simulink model "Model_Comparison"  (R2021a)
settings: Solver=VariableStepAuto  StartTime=0.0  StopTime=3600  RelTol=1e-3
undefined symbols (not defined in the file): A_cell, C1_LUT, Capacity_LUT, Cp_cell, H_cell, M_cell, OCV_LUT, R0_LUT, R1_LUT, SOC_LUT, T_amb, Temperature_LUT
libraries: simulink x1
settings Model: Creator=gopin  LastModifiedBy=gopin

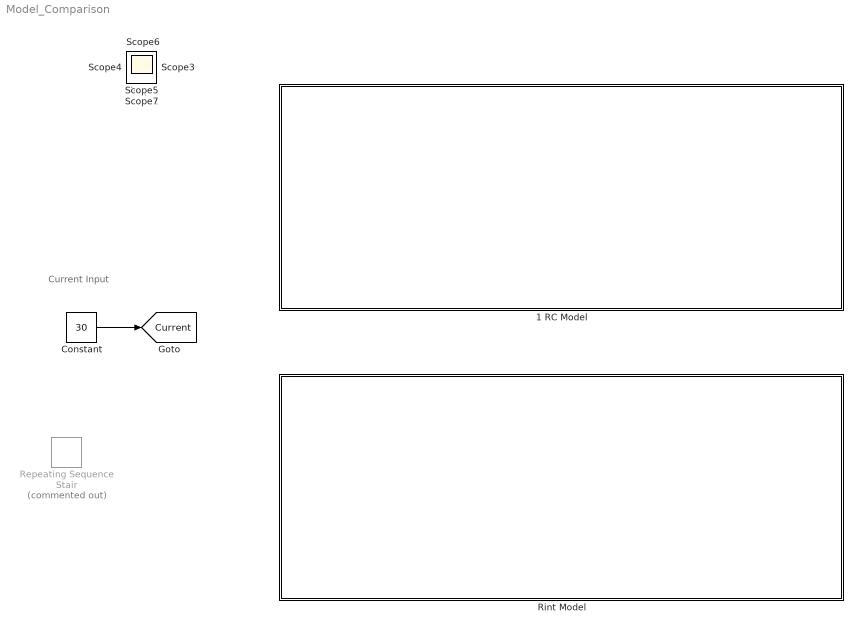
== system Model_Comparison ==
  note: Current Input
  1 RC Model : Subsystem
  Constant : Constant  Value=30
  Repeating Sequence Stair : simulink/Sources/Repeating Sequence Stair  Commented=on  OutValues=[0 0 0 5 9 15 18 18 18 11 8 3 1]  tsamp=-1  OutMin=[]  OutMax=[]  OutDataTypeStr=double  OutputDataTypeScalingMode=double  OutDataType=fixdt(0,8)  ConRadixGroup=Best Precision: Vector-wise  OutScaling=2^-12
  Rint Model : Subsystem
  Scope{,1..7} (8 alike) : Scope
  tag scope: Current=global
  wires:
  Constant/1 -> [Current]

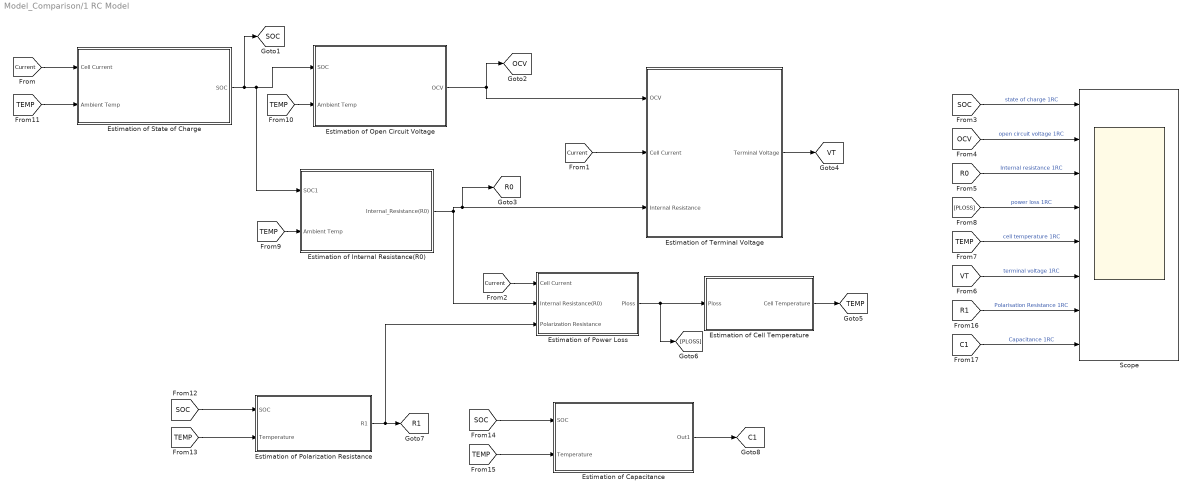
== system Model_Comparison/1 RC Model ==
  Estimation of Capacitance : Subsystem
  Estimation of Cell Temperature : Subsystem
  Estimation of Internal Resistance(R0) : Subsystem
  Estimation of Open Circuit Voltage : Subsystem
  Estimation of Polarization Resistance : Subsystem
  Estimation of Power Loss : Subsystem
  "Estimation of State of Charge " : Subsystem
  Estimation of Terminal Voltage : Subsystem
  Scope : Scope  NumInputPorts=8
  tag scope: C1=global, OCV=global, R0=global, R1=global, SOC=global, TEMP=global, VT=global
  wires:
  Estimation of Terminal Voltage/1(Terminal Voltage) -> [VT]
  [SOC] -> Estimation of Polarization Resistance/1(SOC)
  Estimation of Capacitance/1(Out1) -> [C1]
  [PLOSS] -> Scope/4  "power loss 1RC"
  Estimation of Power Loss/1(Ploss) -> [PLOSS], Estimation of Cell Temperature/1(Ploss)
  [SOC] -> Estimation of Capacitance/1(SOC)
  Estimation of Internal Resistance(R0)/1(Internal_Resistance(R0)) -> [R0], Estimation of Terminal Voltage/3(Internal Resistance), Estimation of Power Loss/2(Internal Resistance(R0))
  [OCV] -> Scope/2  "open circuit voltage 1RC"
  [VT] -> Scope/6  "terminal voltage 1RC"
  [SOC] -> Scope/1  "state of charge 1RC"
  [TEMP] -> Scope/5  "cell temperature 1RC"
  [TEMP] -> Estimation of Capacitance/2(Temperature)
  Estimation of Polarization Resistance/1(R1) -> Estimation of Power Loss/3(Polarization Resistance), [R1]
  [TEMP] -> Estimation of Polarization Resistance/2(Temperature)
  [Current] -> Estimation of Terminal Voltage/2(Cell Current)
  "Estimation of State of Charge "/1(SOC) -> [SOC], Estimation of Internal Resistance(R0)/1(SOC1), Estimation of Open Circuit Voltage/1(SOC)
  Estimation of Open Circuit Voltage/1(OCV) -> Estimation of Terminal Voltage/1(OCV), [OCV]
  [Current] -> Estimation of Power Loss/1(Cell Current)
  [R0] -> Scope/3  "Internal resistance 1RC"
  [TEMP] -> Estimation of Open Circuit Voltage/2(Ambient Temp)
  [Current] -> "Estimation of State of Charge "/1(Cell Current)
  [TEMP] -> Estimation of Internal Resistance(R0)/2(Ambient Temp)
  [TEMP] -> "Estimation of State of Charge "/2(Ambient Temp)
  Estimation of Cell Temperature/1(Cell Temperature) -> [TEMP]
  [R1] -> Scope/7  "Polarisation Resistance 1RC"
  [C1] -> Scope/8  "Capacitance 1RC"

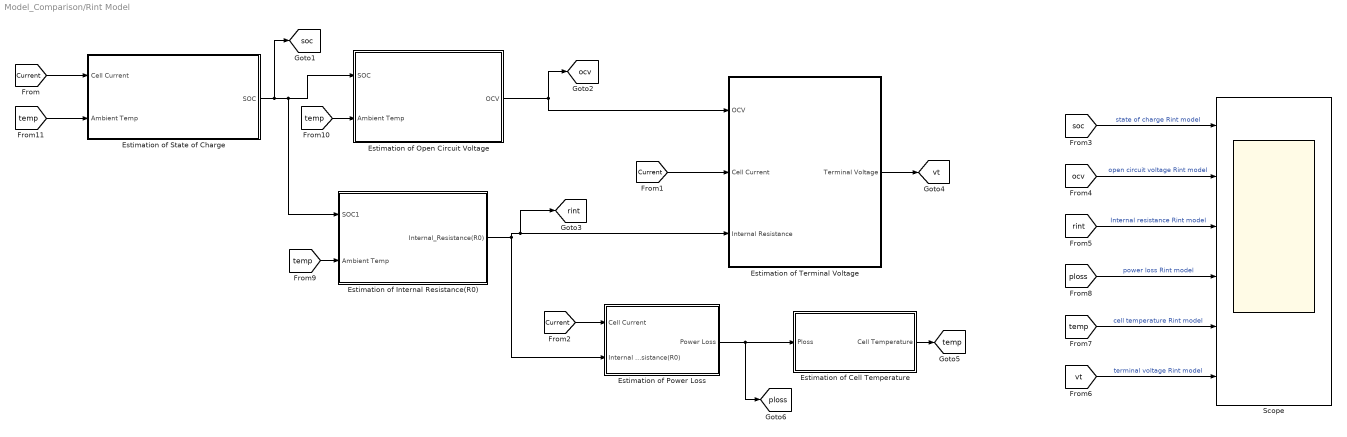
== system Model_Comparison/Rint Model ==
  Estimation of Cell Temperature : Subsystem
  Estimation of Internal Resistance(R0) : Subsystem
  Estimation of Open Circuit Voltage : Subsystem
  Estimation of Power Loss : Subsystem
  "Estimation of State of Charge " : Subsystem
  Estimation of Terminal Voltage : Subsystem
  Scope : Scope  NumInputPorts=6
  tag scope: ocv=global, ploss=global, rint=global, soc=global, temp=global, vt=global
  wires:
  [temp] -> "Estimation of State of Charge "/2(Ambient Temp)
  "Estimation of State of Charge "/1(SOC) -> [soc], Estimation of Internal Resistance(R0)/1(SOC1), Estimation of Open Circuit Voltage/1(SOC)
  [temp] -> Estimation of Internal Resistance(R0)/2(Ambient Temp)
  Estimation of Power Loss/1(Power Loss) -> [ploss], Estimation of Cell Temperature/1(Ploss)
  [Current] -> Estimation of Power Loss/1(Cell Current)
  [rint] -> Scope/3  "Internal resistance Rint model"
  [ocv] -> Scope/2  "open circuit voltage Rint model"
  [temp] -> Scope/5  "cell temperature Rint model"
  [ploss] -> Scope/4  "power loss Rint model"
  Estimation of Cell Temperature/1(Cell Temperature) -> [temp]
  [Current] -> "Estimation of State of Charge "/1(Cell Current)
  Estimation of Internal Resistance(R0)/1(Internal_Resistance(R0)) -> [rint], Estimation of Terminal Voltage/3(Internal Resistance), Estimation of Power Loss/2(Internal Resistance(R0))
  [Current] -> Estimation of Terminal Voltage/2(Cell Current)
  Estimation of Open Circuit Voltage/1(OCV) -> Estimation of Terminal Voltage/1(OCV), [ocv]
  Estimation of Terminal Voltage/1(Terminal Voltage) -> [vt]
  [vt] -> Scope/6  "terminal voltage Rint model"
  [temp] -> Estimation of Open Circuit Voltage/2(Ambient Temp)
  [soc] -> Scope/1  "state of charge Rint model"

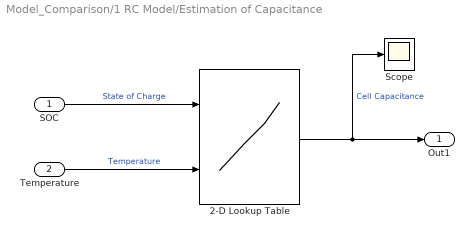
== system Model_Comparison/1 RC Model/Estimation of Capacitance ==
  SOC : Inport
  Temperature : Inport  Port=2
  2-D Lookup Table : Lookup_n-D  BreakpointsForDimension1=SOC_LUT  BreakpointsForDimension2=Temperature_LUT  Table=C1_LUT  InternalRulePriority=Speed  RndMeth=Simplest  InputSameDT=on
      settings: InputPortMap=u0,u1
  Scope : Scope
  Out1 : Outport
  wires:
  SOC/1 -> 2-D Lookup Table/1  "State of Charge"
  Temperature/1 -> 2-D Lookup Table/2  "Temperature"
  2-D Lookup Table/1 -> Scope/1, Out1/1  "Cell Capacitance"

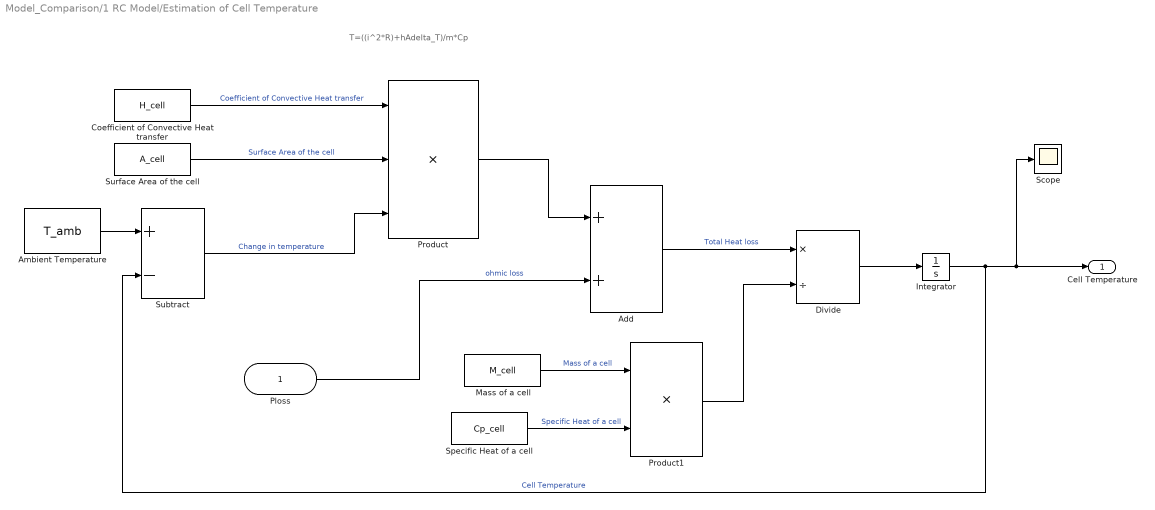
== system Model_Comparison/1 RC Model/Estimation of Cell Temperature ==
  note: T=((i^2*R)+hAdelta_T)/m*Cp
  Ploss : Inport
  Add : Sum
  Ambient Temperature : Constant  Value=T_amb
  Coefficient of Convective Heat transfer : Constant  Value=H_cell
  Divide : Product  Inputs=*/
  Integrator : Integrator  InitialCondition=T_amb  UpperSaturationLimit=353.15  LowerSaturationLimit=T_amb
  Mass of a cell : Constant  Value=M_cell
  Product : Product  Inputs=3
  Product1 : Product
  Scope : Scope
  Specific Heat of a cell : Constant  Value=Cp_cell
  Subtract : Sum  Inputs=+-
  Surface Area of the cell : Constant  Value=A_cell
  Cell Temperature : Outport
  wires:
  Ambient Temperature/1 -> Subtract/1
  Coefficient of Convective Heat transfer/1 -> Product/1  "Coefficient of Convective Heat transfer"
  Surface Area of the cell/1 -> Product/2  "Surface Area of the cell"
  Subtract/1 -> Product/3  "Change in temperature"
  Product/1 -> Add/1
  Ploss/1 -> Add/2  "ohmic loss"
  Add/1 -> Divide/1  "Total Heat loss"
  Product1/1 -> Divide/2
  Mass of a cell/1 -> Product1/1  "Mass of a cell"
  Specific Heat of a cell/1 -> Product1/2  "Specific Heat of a cell"
  Divide/1 -> Integrator/1
  Integrator/1 -> Subtract/2, Scope/1, Cell Temperature/1  "Cell Temperature"

== system Model_Comparison/1 RC Model/Estimation of Internal Resistance(R0) ==
  SOC1 : Inport
  Ambient Temp : Inport  Port=2
  2-D Lookup Table1 : Lookup_n-D  BreakpointsForDimension1=SOC_LUT  BreakpointsForDimension2=Temperature_LUT  Table=R0_LUT  InternalRulePriority=Speed  RndMeth=Simplest  InputSameDT=on
      settings: InputPortMap=u0,u1
  Scope : Scope
  Internal_Resistance(R0) : Outport
  wires:
  SOC1/1 -> 2-D Lookup Table1/1  "state of charge"
  2-D Lookup Table1/1 -> Scope/1, Internal_Resistance(R0)/1  "Internal Resistance"
  Ambient Temp/1 -> 2-D Lookup Table1/2  "Ambient Temperature"

== system Model_Comparison/1 RC Model/Estimation of Open Circuit Voltage ==
  SOC : Inport
  Ambient Temp : Inport  Port=2
  2-D Lookup Table : Lookup_n-D  BreakpointsForDimension1=SOC_LUT  BreakpointsForDimension2=Temperature_LUT  Table=OCV_LUT  InternalRulePriority=Speed  RndMeth=Simplest  InputSameDT=on
      settings: InputPortMap=u0,u1
  Scope : Scope
  OCV : Outport
  wires:
  SOC/1 -> 2-D Lookup Table/1  "state of charge"
  2-D Lookup Table/1 -> Scope/1, OCV/1  "open circuit voltage"
  Ambient Temp/1 -> 2-D Lookup Table/2  "Ambient Temperature"

== system Model_Comparison/1 RC Model/Estimation of Polarization Resistance ==
  SOC : Inport
  Temperature : Inport  Port=2
  2-D Lookup Table : Lookup_n-D  BreakpointsForDimension1=SOC_LUT  BreakpointsForDimension2=Temperature_LUT  Table=R1_LUT  InternalRulePriority=Speed  RndMeth=Simplest  InputSameDT=on
      settings: InputPortMap=u0,u1
  Scope : Scope
  R1 : Outport
  wires:
  SOC/1 -> 2-D Lookup Table/1  "State of Charge"
  Temperature/1 -> 2-D Lookup Table/2  "Temperature"
  2-D Lookup Table/1 -> Scope/1, R1/1  "Polarization Resistance"

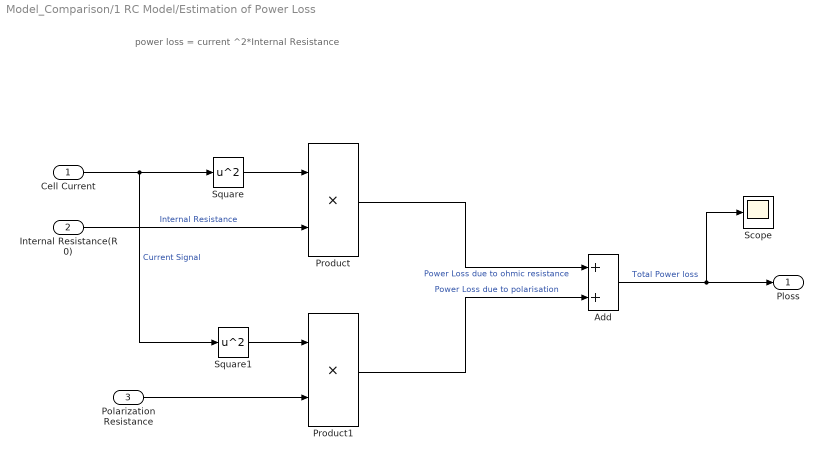
== system Model_Comparison/1 RC Model/Estimation of Power Loss ==
  note: power loss = current ^2*Internal Resistance
  Cell Current : Inport
  Internal Resistance(R0) : Inport  Port=2
  Polarization Resistance : Inport  Port=3
  Add : Sum
  Product : Product
  Product1 : Product
  Scope : Scope
  Square : Math  Operator=square  SaturateOnIntegerOverflow=on
  Square1 : Math  Operator=square  SaturateOnIntegerOverflow=on
  Ploss : Outport
  wires:
  Cell Current/1 -> Square1/1, Square/1  "Current Signal"
  Square/1 -> Product/1
  Product/1 -> Add/1  "Power Loss due to ohmic resistance"
  Internal Resistance(R0)/1 -> Product/2  "Internal Resistance"
  Square1/1 -> Product1/1
  Polarization Resistance/1 -> Product1/2
  Product1/1 -> Add/2  "Power Loss due to polarisation"
  Add/1 -> Scope/1, Ploss/1  "Total Power loss"

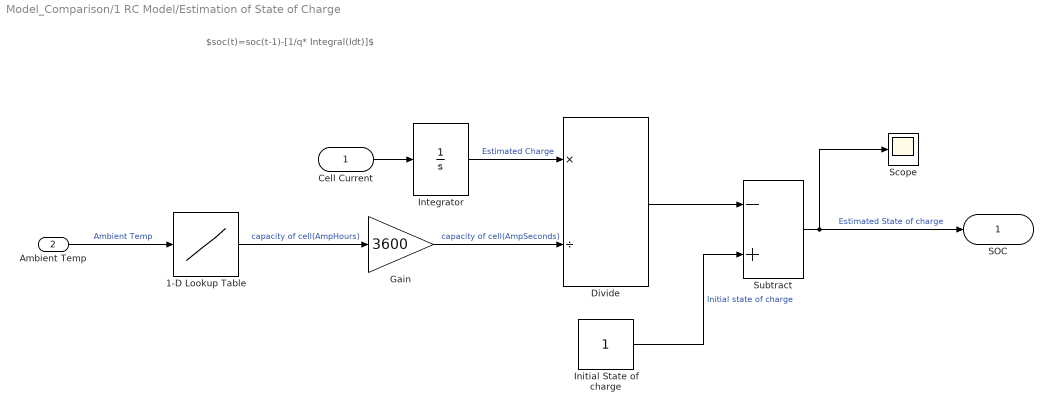
== system Model_Comparison/1 RC Model/Estimation of State of Charge  ==
  note: $soc(t)=soc(t-1)-[1/q* Integral(Idt)]$
  Cell Current : Inport
  Ambient Temp : Inport  Port=2
  1-D Lookup Table : Lookup_n-D  NumberOfTableDimensions=1  BreakpointsForDimension1=Temperature_LUT  Table=Capacity_LUT  InternalRulePriority=Speed  RndMeth=Simplest  InputSameDT=on
  Divide : Product  Inputs=*/
  Gain : Gain  Gain=3600
  Initial State of charge : Constant
  Integrator : Integrator
  Scope : Scope
  Subtract : Sum  Inputs=-+
  SOC : Outport
  wires:
  Initial State of charge/1 -> Subtract/2  "Initial state of charge"
  Subtract/1 -> Scope/1, SOC/1  "Estimated State of charge"
  Integrator/1 -> Divide/1  "Estimated Charge"
  Divide/1 -> Subtract/1
  Cell Current/1 -> Integrator/1
  1-D Lookup Table/1 -> Gain/1  "capacity of cell(AmpHours)"
  Gain/1 -> Divide/2  "capacity of cell(AmpSeconds)"
  Ambient Temp/1 -> 1-D Lookup Table/1  "Ambient Temp"

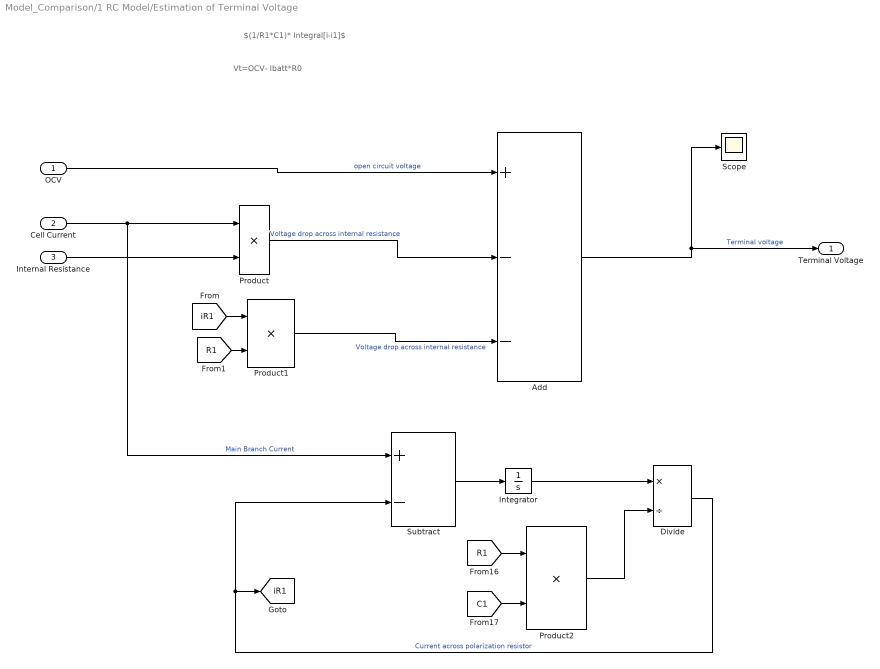
== system Model_Comparison/1 RC Model/Estimation of Terminal Voltage ==
  note: Vt=OCV- Ibatt*R0
  note: $(1/R1*C1)* Integral[i-i1]$
  OCV : Inport
  Cell Current : Inport  Port=2
  Internal Resistance : Inport  Port=3
  Add : Sum  Inputs=+--
  Divide : Product  Inputs=*/
  Integrator : Integrator
  Product : Product
  Product1 : Product
  Product2 : Product
  Scope : Scope
  Subtract : Sum  Inputs=+-
  Terminal Voltage : Outport
  tag scope: iR1=global
  wires:
  Add/1 -> Scope/1, Terminal Voltage/1  "Terminal voltage"
  OCV/1 -> Add/1  "open circuit voltage"
  Product/1 -> Add/2  "Voltage drop across internal resistance"
  Cell Current/1 -> Subtract/1, Product/1  "Main Branch Current"
  Internal Resistance/1 -> Product/2
  Product1/1 -> Add/3  "Voltage drop across internal resistance"
  Divide/1 -> [iR1], Subtract/2  "Current across polarization resistor"
  Subtract/1 -> Integrator/1
  Integrator/1 -> Divide/1
  Product2/1 -> Divide/2
  [R1] -> Product2/1
  [C1] -> Product2/2
  [iR1] -> Product1/1
  [R1] -> Product1/2

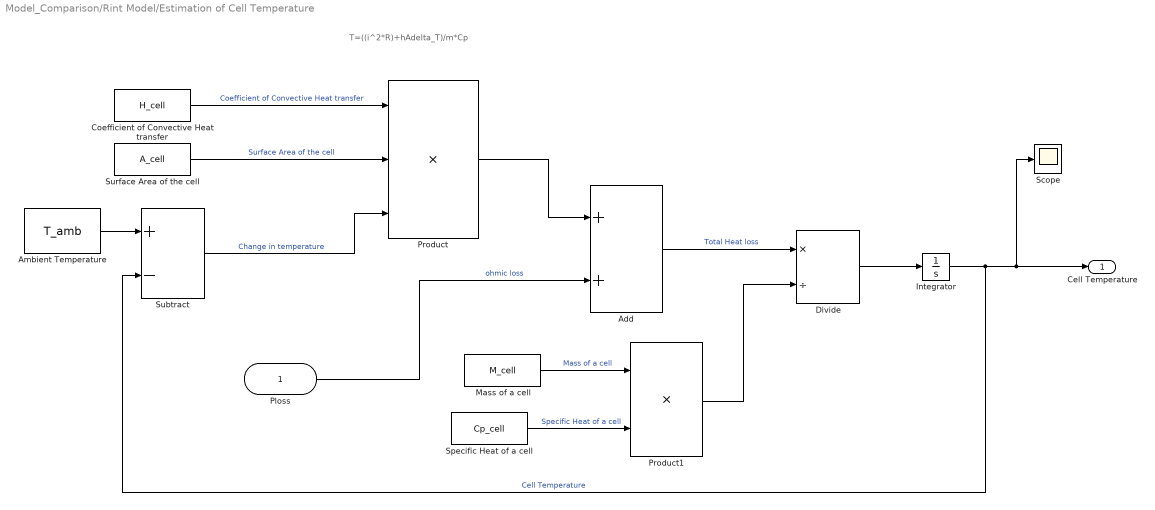
== system Model_Comparison/Rint Model/Estimation of Cell Temperature ==
  note: T=((i^2*R)+hAdelta_T)/m*Cp
  Ploss : Inport
  Add : Sum
  Ambient Temperature : Constant  Value=T_amb
  Coefficient of Convective Heat transfer : Constant  Value=H_cell
  Divide : Product  Inputs=*/
  Integrator : Integrator  InitialCondition=T_amb  UpperSaturationLimit=353.15  LowerSaturationLimit=T_amb
  Mass of a cell : Constant  Value=M_cell
  Product : Product  Inputs=3
  Product1 : Product
  Scope : Scope
  Specific Heat of a cell : Constant  Value=Cp_cell
  Subtract : Sum  Inputs=+-
  Surface Area of the cell : Constant  Value=A_cell
  Cell Temperature : Outport
  wires:
  Ambient Temperature/1 -> Subtract/1
  Coefficient of Convective Heat transfer/1 -> Product/1  "Coefficient of Convective Heat transfer"
  Surface Area of the cell/1 -> Product/2  "Surface Area of the cell"
  Subtract/1 -> Product/3  "Change in temperature"
  Product/1 -> Add/1
  Ploss/1 -> Add/2  "ohmic loss"
  Add/1 -> Divide/1  "Total Heat loss"
  Product1/1 -> Divide/2
  Mass of a cell/1 -> Product1/1  "Mass of a cell"
  Specific Heat of a cell/1 -> Product1/2  "Specific Heat of a cell"
  Divide/1 -> Integrator/1
  Integrator/1 -> Subtract/2, Scope/1, Cell Temperature/1  "Cell Temperature"

== system Model_Comparison/Rint Model/Estimation of Internal Resistance(R0) ==
  SOC1 : Inport
  Ambient Temp : Inport  Port=2
  2-D Lookup Table1 : Lookup_n-D  BreakpointsForDimension1=SOC_LUT  BreakpointsForDimension2=Temperature_LUT  Table=R0_LUT  InternalRulePriority=Speed  RndMeth=Simplest  InputSameDT=on
      settings: InputPortMap=u0,u1
  Scope : Scope
  Internal_Resistance(R0) : Outport
  wires:
  SOC1/1 -> 2-D Lookup Table1/1  "state of charge"
  2-D Lookup Table1/1 -> Scope/1, Internal_Resistance(R0)/1  "Internal Resistance"
  Ambient Temp/1 -> 2-D Lookup Table1/2  "Ambient Temperature"

== system Model_Comparison/Rint Model/Estimation of Open Circuit Voltage ==
  SOC : Inport
  Ambient Temp : Inport  Port=2
  2-D Lookup Table : Lookup_n-D  BreakpointsForDimension1=SOC_LUT  BreakpointsForDimension2=Temperature_LUT  Table=OCV_LUT  InternalRulePriority=Speed  RndMeth=Simplest  InputSameDT=on
      settings: InputPortMap=u0,u1
  Scope : Scope
  OCV : Outport
  wires:
  SOC/1 -> 2-D Lookup Table/1  "state of charge"
  2-D Lookup Table/1 -> Scope/1, OCV/1  "open circuit voltage"
  Ambient Temp/1 -> 2-D Lookup Table/2  "Ambient Temperature"

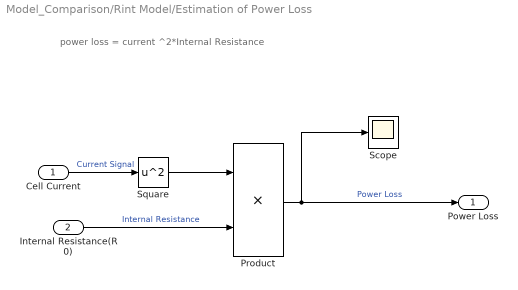
== system Model_Comparison/Rint Model/Estimation of Power Loss ==
  note: power loss = current ^2*Internal Resistance
  Cell Current : Inport
  Internal Resistance(R0) : Inport  Port=2
  Product : Product
  Scope : Scope
  Square : Math  Operator=square  SaturateOnIntegerOverflow=on
  Power Loss : Outport
  wires:
  Cell Current/1 -> Square/1  "Current Signal"
  Square/1 -> Product/1
  Product/1 -> Scope/1, Power Loss/1  "Power Loss"
  Internal Resistance(R0)/1 -> Product/2  "Internal Resistance"

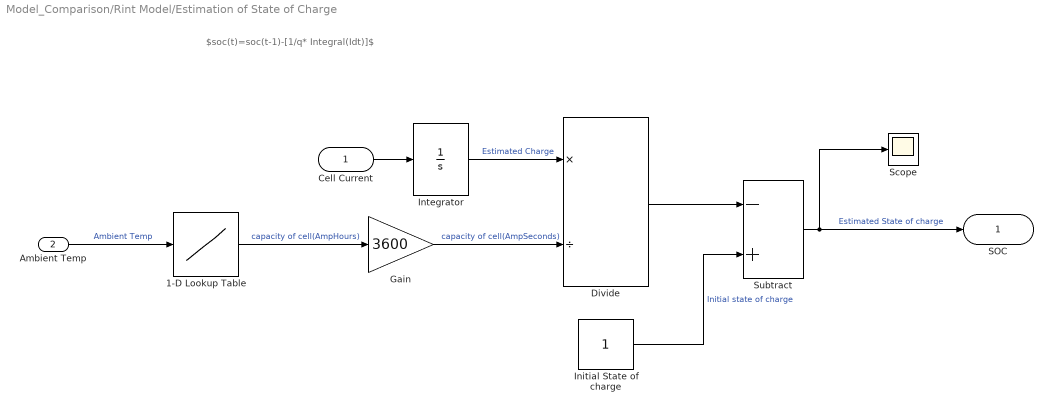
== system Model_Comparison/Rint Model/Estimation of State of Charge  ==
  note: $soc(t)=soc(t-1)-[1/q* Integral(Idt)]$
  Cell Current : Inport
  Ambient Temp : Inport  Port=2
  1-D Lookup Table : Lookup_n-D  NumberOfTableDimensions=1  BreakpointsForDimension1=Temperature_LUT  Table=Capacity_LUT  InternalRulePriority=Speed  RndMeth=Simplest  InputSameDT=on
  Divide : Product  Inputs=*/
  Gain : Gain  Gain=3600
  Initial State of charge : Constant
  Integrator : Integrator
  Scope : Scope
  Subtract : Sum  Inputs=-+
  SOC : Outport
  wires:
  Initial State of charge/1 -> Subtract/2  "Initial state of charge"
  Subtract/1 -> Scope/1, SOC/1  "Estimated State of charge"
  Integrator/1 -> Divide/1  "Estimated Charge"
  Divide/1 -> Subtract/1
  Cell Current/1 -> Integrator/1
  1-D Lookup Table/1 -> Gain/1  "capacity of cell(AmpHours)"
  Gain/1 -> Divide/2  "capacity of cell(AmpSeconds)"
  Ambient Temp/1 -> 1-D Lookup Table/1  "Ambient Temp"

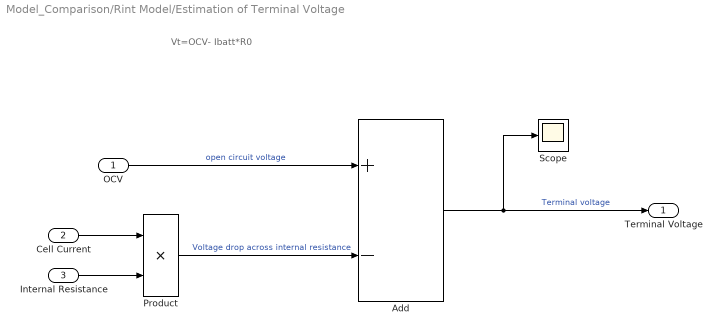
== system Model_Comparison/Rint Model/Estimation of Terminal Voltage ==
  note: Vt=OCV- Ibatt*R0
  OCV : Inport
  Cell Current : Inport  Port=2
  Internal Resistance : Inport  Port=3
  Add : Sum  Inputs=+-
  Product : Product
  Scope : Scope
  Terminal Voltage : Outport
  wires:
  Add/1 -> Scope/1, Terminal Voltage/1  "Terminal voltage"
  OCV/1 -> Add/1  "open circuit voltage"
  Product/1 -> Add/2  "Voltage drop across internal resistance"
  Cell Current/1 -> Product/1
  Internal Resistance/1 -> Product/2
